simulink library "Valeo_Simulink_Library_EC"  (R2017b)
settings: Solver=ode45  StartTime=0.0  StopTime=10.0  RelTol=1e-3  EnableMultiTasking=on
undefined symbols (not defined in the file or in its folder): A, B, C, Count_Max, D, InitValue, j, ke, kf, kt, L, Length, MaxIniVal, MaxVal, MinVal, NumBits1, NumBits2, P, p0, Q, R, Simulink_Library, Ts, x0
libraries: Valeo_Simulink_Library_EC x9, simulink x4, fixpt_dtprop x4
(part 4 of 4)

== system Valeo_Simulink_Library_EC/Plant Models/Actuators/BLDC/BLDC motor Block/Trapz_f ==
  note: sinusoidal BEMF
  note: Instead of Position range: 0-5, output can be mapped to HALL sensor readings,
      | then inverter logic must be changed accordingly!
  Theta_m : Inport
  1-D Lookup Table : Lookup_n-D  NumberOfTableDimensions=1  BreakpointsForDimension1=0:pi/3:2*pi  Table=[1 1 1 -1 -1 -1 1]  RndMeth=Simplest  InputSameDT=on
  1-D Lookup Table1 : Lookup_n-D  NumberOfTableDimensions=1  BreakpointsForDimension1=0:pi/3:2*pi  Table=[-1 -1 1 1 1 -1 -1]  RndMeth=Simplest  InputSameDT=on
  1-D Lookup Table2 : Lookup_n-D  NumberOfTableDimensions=1  BreakpointsForDimension1=0:pi/3:2*pi  Table=[1 -1 -1 -1 1 1 1]  RndMeth=Simplest  InputSameDT=on
  1-D Lookup Table3 : Lookup_n-D  NumberOfTableDimensions=1  BreakpointsForDimension1=[0 1.047 pi/3 2.0942 2*pi/3 3.1414 pi 4.1886 4*pi/3 5.2358 5*pi/3 6.283 ]  Table=[0 0 1 1 2 2 3 3 4 4 5 5]  TableDataTypeStr=uint8  ExtrapMethod=Clip  OutDataTypeStr=uint8  RndMeth=Simplest  InputSameDT=on
  Fcn : Fcn  Expr=rem(u,2*pi)
  Gain : Gain  Gain=P/2
  Manual Switch : ManualSwitch  CurrentSetting=0
  Mux : Mux  Inputs=3
  Mux1 : Mux  Inputs=3
  Scope : Scope
  Sine Wave : Sin  TimeSource=Use external signal  SampleTime=0
  Sine Wave1 : Sin  TimeSource=Use external signal  Phase=-2*pi/3  SampleTime=0
  Sine Wave2 : Sin  TimeSource=Use external signal  Phase=-4*pi/3  SampleTime=0
  Position : Outport  VectorParamsAs1DForOutWhenUnconnected=off
  f_abc : Outport  Port=2  VectorParamsAs1DForOutWhenUnconnected=off
  wires:
  Theta_m/1 -> Gain/1
  Gain/1 -> Fcn/1
  1-D Lookup Table/1 -> Mux/1
  1-D Lookup Table1/1 -> Mux/2
  1-D Lookup Table2/1 -> Mux/3
  Mux/1 -> Manual Switch/2  "trapz"
  Fcn/1 -> 1-D Lookup Table3/1, 1-D Lookup Table2/1, 1-D Lookup Table/1, Sine Wave/1, Sine Wave1/1, Sine Wave2/1, 1-D Lookup Table1/1  "Theta_e"
  1-D Lookup Table3/1 -> Position/1
  Sine Wave2/1 -> Mux1/3
  Sine Wave1/1 -> Mux1/2
  Sine Wave/1 -> Mux1/1
  Mux1/1 -> Manual Switch/1  "sin"
  Manual Switch/1 -> Scope/1, f_abc/1

== stateflow chart Valeo_Simulink_Library_EC/Math_Operations/VSL_DynamicSecureDivision_EC_Blk/Calculation/DecisionLogic/DynamicSecureDivision ==
  settings: description=this block is performing secure division with Positive_inf, Negative_inf, Nan is dynamic in run time
  (default) -> (junction 8)
  (junction 8) -> (junction 9) [order 1] : [abs(Den)<=ZeroBand_Den]
  (junction 8) -> (junction 14) [order 2]
  (junction 9) -> (junction 58)
  (junction 14) -> (junction 16) [order 1] : [abs(Num)<=ZeroBand_Num]
  (junction 58) -> (junction 60) [order 1] : [abs(Num)<=ZeroBand_Num]
  (junction 14) -> (junction 26) [order 2] : {
      | Divide;
      | }
  (junction 16) -> (junction 67) : {
      | Output = 0;
      | }
  (junction 58) -> (junction 18) [order 2]
  (junction 60) -> (junction 61) : {
      | Output = Nan;
      | }
  (junction 18) -> (junction 20) [order 1] : [Num>0]
  (junction 18) -> (junction 24) [order 2] : {
      | Output = Negative_Inf;
      | }
  (junction 20) -> (junction 22) : {
      | Output = Positive_Inf;
      | }
  (junction 67) -> (junction 26)
  (junction 24) -> (junction 67)
  (junction 22) -> (junction 24)
  (junction 61) -> (junction 22)
  (junction 26) -> (junction 31)
  data: Num input; Den input; Positive_Inf input; Negative_Inf input; Nan input; Output output; ZeroBand_Den input; ZeroBand_Num input
  events: Divide output FUNCTION_CALL_EVENT

== matlab function Valeo_Simulink_Library_EC/Plant Models/Actuators/BLDC/inverter/MATLAB Function ==
  data: POS input; Vs input; e_abc input; U output; i_abc input
function U = inverter(POS,Vs,e_abc,i_abc)
%U: [Vab-Eab;Vbc-Ebc]
ebs=0.00000001;% comparing to zero destabilize the solver

if (POS==0) && (i_abc(3)>ebs) 
U= [Vs-e_abc(1)+e_abc(2);-e_abc(2)+e_abc(3)];
elseif  (POS==0) && (i_abc(3)<=ebs)
U= [Vs-e_abc(1)+e_abc(2);0.5*(-Vs+e_abc(1)-e_abc(2))];

elseif (POS==1) && (i_abc(2)<ebs)
U= [-e_abc(1)+e_abc(2);Vs-e_abc(2)+e_abc(3)];
elseif  (POS==1) && (i_abc(2)>=ebs)
U= [0.5*(Vs-e_abc(1)+e_abc(3));0.5*(Vs-e_abc(1)+e_abc(3))];

elseif (POS==2) && (i_abc(1)>ebs)
U= [-Vs-e_abc(1)+e_abc(2);Vs-e_abc(2)+e_abc(3)];
elseif  (POS==2) && (i_abc(1)<=ebs)
U= [0.5*(-Vs+e_abc(2)-e_abc(3));Vs-e_abc(2)+e_abc(3)];

elseif (POS==3)&& (i_abc(3)<ebs)
U= [-Vs-e_abc(1)+e_abc(2);-e_abc(2)+e_abc(3)];
elseif  (POS==3) && (i_abc(3)>=ebs)
U= [-Vs-e_abc(1)+e_abc(2);0.5*(Vs+e_abc(1)-e_abc(2))];

elseif (POS==4) && (i_abc(2)>ebs)
U= [-e_abc(1)+e_abc(2);-Vs-e_abc(2)+e_abc(3)];
elseif   (POS==4) && (i_abc(2)<=ebs)
U= [0.5*(-Vs-e_abc(1)+e_abc(3));0.5*(-Vs-e_abc(1)+e_abc(3))];

elseif (POS==5) && (i_abc(1)<ebs)
U= [Vs-e_abc(1)+e_abc(2);-Vs-e_abc(2)+e_abc(3)];
elseif   (POS==5) && (i_abc(1)>=ebs)
U= [0.5*(Vs+e_abc(2)-e_abc(3));-Vs-e_abc(2)+e_abc(3)];

 else
 U=[0.0;0.0]; % has no contribution to calculation , but it must be included as a work around to an error of 
end
